simulink model "exer3_1"  (R2014b)
settings: Solver=ode45  StartTime=0.0  StopTime=2  RelTol=1e-3
libraries: simulink x1
settings Model: Creator=Charlie  LastModifiedBy=Charlie

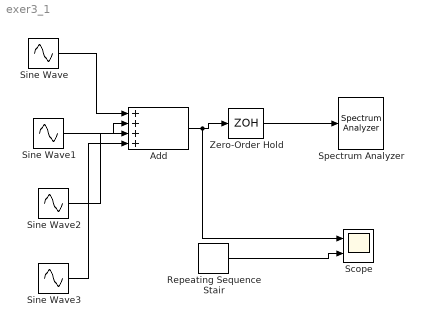
== system exer3_1 ==
  Add : Sum  Inputs=++++
  Repeating Sequence Stair : simulink/Sources/Repeating Sequence Stair  OutValues=[1 -1]  tsamp=1/64  OutMin=[]  OutMax=[]  OutDataTypeStr=double  OutputDataTypeScalingMode=double  OutDataType=fixdt(0,8)  ConRadixGroup=Best Precision: Vector-wise  OutScaling=2^-12
  Scope : Scope  NumInputPorts=2
      settings: YMin=-5~-5  YMax=5~5
  Sine Wave : Sin  Amplitude=0.112  Frequency=1407.4  SampleTime=0
  Sine Wave1 : Sin  Amplitude=0.7854  Frequency=201.062  SampleTime=0
  Sine Wave2 : Sin  Amplitude=0.262  Frequency=603.2  SampleTime=0
  Sine Wave3 : Sin  Amplitude=0.157  Frequency=1005.3  SampleTime=0
  Spectrum Analyzer : SpectrumAnalyzer
  Zero-Order Hold : ZeroOrderHold  SampleTime=2e-5
  wires:
  Sine Wave/1 -> Add/1
  Sine Wave1/1 -> Add/2
  Sine Wave2/1 -> Add/3
  Sine Wave3/1 -> Add/4
  Add/1 -> Scope/1, Zero-Order Hold/1
  Zero-Order Hold/1 -> Spectrum Analyzer/1
  Repeating Sequence Stair/1 -> Scope/2
